simulink subsystem "CustomDualFFT"  (R2024b)
settings: Solver=VariableStepAuto  StartTime=0.0  StopTime=10.0  RelTol=1e-3
settings Model: Creator=JesseJabezArendse  LastModifiedBy=JesseJabezArendse
settings RTWCC: GPUComputeCapability=3.5

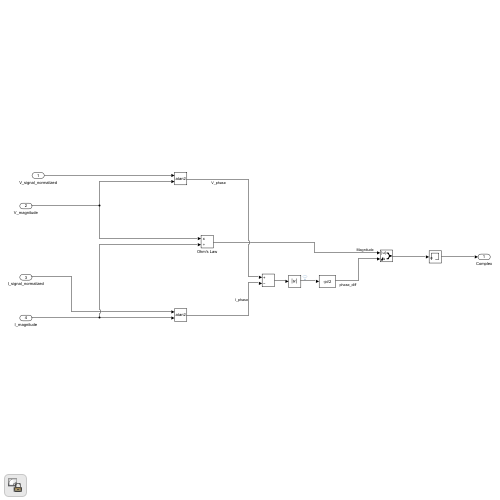
[thumbnail: Simulink's stored preview of the top-level diagram]
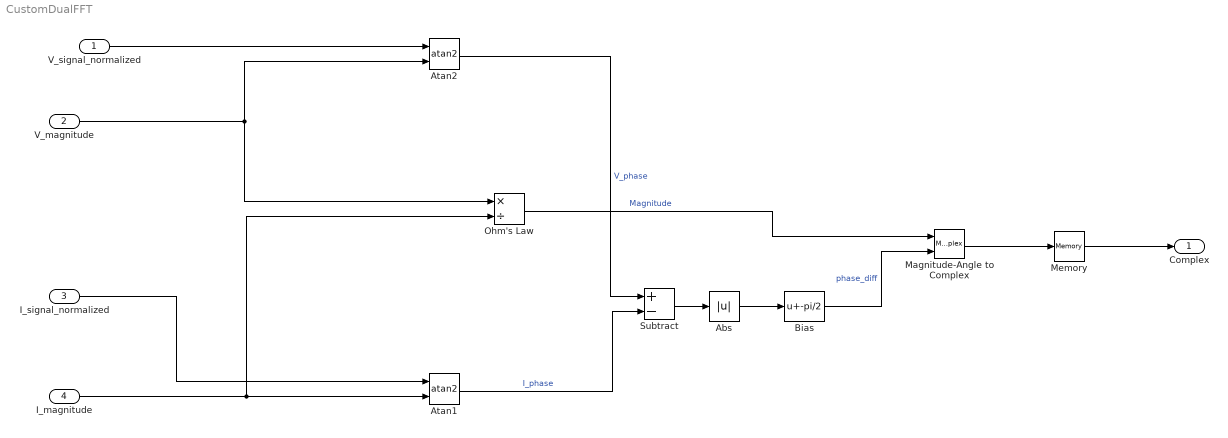
== system CustomDualFFT ==
  V_signal_normalized : Inport  OutDataTypeStr=single
  V_magnitude : Inport  Port=2
  I_signal_normalized : Inport  Port=3  OutDataTypeStr=single
  I_magnitude : Inport  Port=4
  Abs : Abs  OutDataTypeStr=single  SaturateOnIntegerOverflow=off
  Atan1 : Trigonometry  Operator=atan2  OutputSignalType=real
  Atan2 : Trigonometry  Operator=atan2  OutputSignalType=real
  Bias : Bias  Bias=-pi/2  SaturateOnIntegerOverflow=off
  Magnitude-Angle to Complex : MagnitudeAngleToComplex
  Memory : Memory  InheritSampleTime=on
  Ohm's Law : Product  Inputs=*/  OutDataTypeStr=single
  Subtract : Sum  Inputs=+-  OutDataTypeStr=single
  Complex : Outport
  wires:
  Memory/1 -> Complex/1
  Magnitude-Angle to Complex/1 -> Memory/1
  Atan1/1 -> Subtract/2  "I_phase"
  Atan2/1 -> Subtract/1  "V_phase"
  Subtract/1 -> Abs/1
  Abs/1 -> Bias/1
  Ohm's Law/1 -> Magnitude-Angle to Complex/1  "Magnitude"
  V_signal_normalized/1 -> Atan2/1
  V_magnitude/1 -> Ohm's Law/1, Atan2/2
  I_signal_normalized/1 -> Atan1/1
  I_magnitude/1 -> Ohm's Law/2, Atan1/2
  Bias/1 -> Magnitude-Angle to Complex/2  "phase_diff"
